simulink model "gm_IPCore_3Level_PWM"  (R2025b)
settings: Solver=VariableStepAuto  StartTime=0.0  StopTime=0.01  RelTol=1e-3
undefined symbols (not defined in the file or in its folder): f_Carrier, f_FPGA_clk, T_FPGA_clk
libraries: hdlsllib x3
settings Model: Creator=info  LastModifiedBy=info
settings OptimizationCC: BlockReduction=off  ConditionallyExecuteInputs=off  DefaultParameterBehavior=Inlined
settings DebuggingCC: AlgebraicLoopMsg=error  InheritedTsInSrcMsg=none  SingleTaskRateTransMsg=error
settings HardwareCC: ProdBitPerPointer=32.0  ProdBitPerSizeT=32.0  ProdBitPerPtrDiffT=32.0  ProdLargestAtomicFloat=None  ProdIntDivRoundTo=Undefined  ProdEndianess=Unspecified  ProdWordSize=32.0  ProdHWDeviceType=ASIC/FPGA->ASIC/FPGA  TargetBitPerPointer=64.0  TargetBitPerSizeT=64.0  TargetBitPerPtrDiffT=64.0  TargetLongLongMode=on  TargetIntDivRoundTo=Zero  TargetEndianess=LittleEndian  TargetWordSize=64.0  TargetHWDeviceType=Custom Processor->MATLAB Host Computer  ProdEqTarget=off

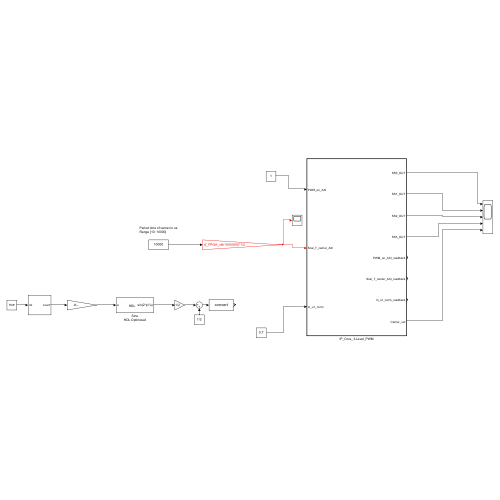
[thumbnail: Simulink's stored preview of the top-level diagram]
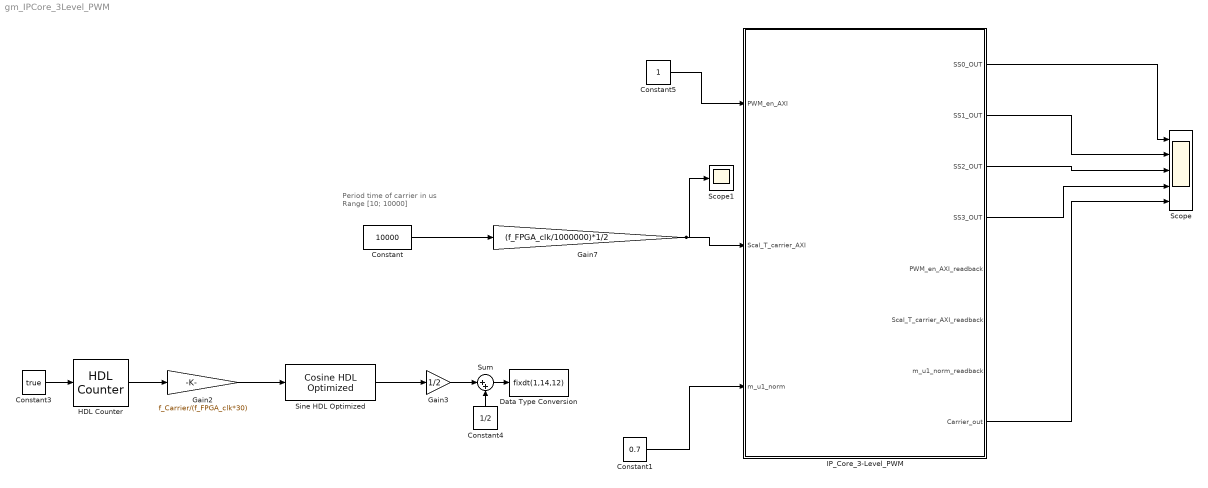
== system gm_IPCore_3Level_PWM ==
  note: Period time of carrier in us
      | Range [10; 10000]
  Constant : Constant  Value=10000  SampleTime=T_FPGA_clk
  Constant1 : Constant  Value=0.7  OutDataTypeStr=fixdt(1,14,12)  SampleTime=T_FPGA_clk
  Constant3 : Constant  Value=true  OutDataTypeStr=boolean  SampleTime=T_FPGA_clk
  Constant4 : Constant  Value=1/2  SampleTime=-1
  Constant5 : Constant  OutDataTypeStr=boolean  SampleTime=T_FPGA_clk
  Data Type Conversion : DataTypeConversion  OutDataTypeStr=fixdt(1,14,12)  SaturateOnIntegerOverflow=off  RndMeth=Floor
  Gain2 : Gain  Gain=f_Carrier/(f_FPGA_clk*30)
  Gain3 : Gain  Gain=1/2
  Gain7 : Gain  Gain=(f_FPGA_clk/1000000)*1/2  OutDataTypeStr=fixdt(0,25,0)
  HDL Counter : hdlsllib/Sources/HDL Counter  CountType=Free running  CountInit=0  CountStep=1  CountMax=25  CountFromType=Initial value  CountFrom=0  CountResetPort=off  CountLoadPort=off  CountEnbPort=off  CountDirPort=on  CountHitOutputPort=off  CountDataType=Unsigned  CountWordLen=20  CountFracLen=0  CountSampTime=1
  IP_Core_3-Level_PWM : Subsystem  TreatAsAtomicUnit=on
  Scope : Scope  NumInputPorts=5
      settings: ActiveDisplayYMinimum=-0.12499999999999997  ActiveDisplayYMaximum=1.125  DataLoggingVariableName=ScopeData2  DataLoggingSaveFormat=Array
  Scope1 : Scope
      settings: ActiveDisplayYMinimum=-2.0551334999999995E+6  ActiveDisplayYMaximum=1.85012015E+7  DataLoggingSaveFormat=Array
  Sine HDL Optimized : hdlsllib/Lookup Tables/Cosine HDL Optimized  OutputFormula=sin(2*pi*u)  NumDataPoints=64  TableDataTypeStr=fixdt(0,16,15)  SimulateLUTROMDelay=off
      settings: LibrarySourceBlock=|
      | hdlsllib/Lookup
      | Tables/Sine
      | HDL Optimized
  Sum : Sum  Inputs=|++
  wires:
  IP_Core_3-Level_PWM/8(Carrier_out) -> Scope/5
  Constant1/1 -> IP_Core_3-Level_PWM/3(m_u1_norm)
  IP_Core_3-Level_PWM/4(SS3_OUT) -> Scope/4
  IP_Core_3-Level_PWM/3(SS2_OUT) -> Scope/3
  IP_Core_3-Level_PWM/2(SS1_OUT) -> Scope/2
  IP_Core_3-Level_PWM/1(SS0_OUT) -> Scope/1
  Constant5/1 -> IP_Core_3-Level_PWM/1(PWM_en_AXI)
  Sum/1 -> Data Type Conversion/1
  Gain3/1 -> Sum/1
  Constant4/1 -> Sum/2
  Constant3/1 -> HDL Counter/1
  HDL Counter/1 -> Gain2/1
  Gain2/1 -> Sine HDL Optimized/1
  Sine HDL Optimized/1 -> Gain3/1
  Gain7/1 -> IP_Core_3-Level_PWM/2(Scal_T_carrier_AXI), Scope1/1
  Constant/1 -> Gain7/1

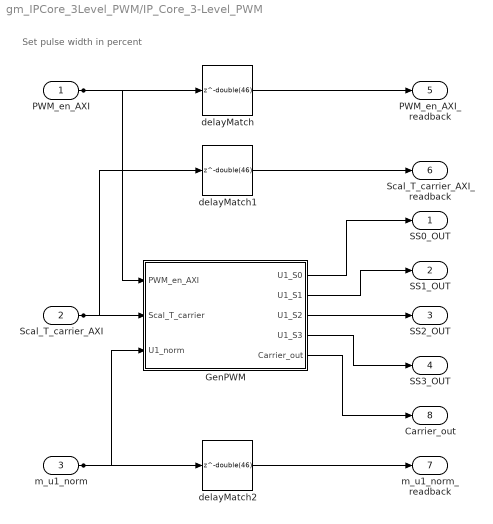
== system gm_IPCore_3Level_PWM/IP_Core_3-Level_PWM ==
  note: Set pulse width in percent
  PWM_en_AXI : Inport  OutDataTypeStr=boolean  PortDimensions=1  SampleTime=1e-08
  Scal_T_carrier_AXI : Inport  Port=2  OutDataTypeStr=fixdt(0, 25, 0)  PortDimensions=1  SampleTime=1e-08
  m_u1_norm : Inport  Port=3  OutDataTypeStr=fixdt(1, 14, 12)  PortDimensions=1  SampleTime=1e-08
  GenPWM : Subsystem
  delayMatch : Delay  DelayLength=double(46)  InitialCondition=0  SampleTime=1e-08
  delayMatch1 : Delay  DelayLength=double(46)  InitialCondition=0  SampleTime=1e-08
  delayMatch2 : Delay  DelayLength=double(46)  InitialCondition=0  SampleTime=1e-08
  SS0_OUT : Outport  SampleTime=1e-08  VectorParamsAs1DForOutWhenUnconnected=off
  SS1_OUT : Outport  Port=2  SampleTime=1e-08  VectorParamsAs1DForOutWhenUnconnected=off
  SS2_OUT : Outport  Port=3  SampleTime=1e-08  VectorParamsAs1DForOutWhenUnconnected=off
  SS3_OUT : Outport  Port=4  SampleTime=1e-08  VectorParamsAs1DForOutWhenUnconnected=off
  PWM_en_AXI_readback : Outport  Port=5  SampleTime=1e-08  VectorParamsAs1DForOutWhenUnconnected=off
  Scal_T_carrier_AXI_readback : Outport  Port=6  SampleTime=1e-08
  m_u1_norm_readback : Outport  Port=7  SampleTime=1e-08
  Carrier_out : Outport  Port=8  SampleTime=1e-08
  wires:
  PWM_en_AXI/1 -> GenPWM/1(PWM_en_AXI), delayMatch/1
  Scal_T_carrier_AXI/1 -> delayMatch1/1, GenPWM/2(Scal_T_carrier)
  delayMatch1/1 -> Scal_T_carrier_AXI_readback/1
  m_u1_norm/1 -> delayMatch2/1, GenPWM/3(U1_norm)
  delayMatch2/1 -> m_u1_norm_readback/1
  delayMatch/1 -> PWM_en_AXI_readback/1
  GenPWM/1(U1_S0) -> SS0_OUT/1
  GenPWM/2(U1_S1) -> SS1_OUT/1
  GenPWM/3(U1_S2) -> SS2_OUT/1
  GenPWM/4(U1_S3) -> SS3_OUT/1
  GenPWM/5(Carrier_out) -> Carrier_out/1

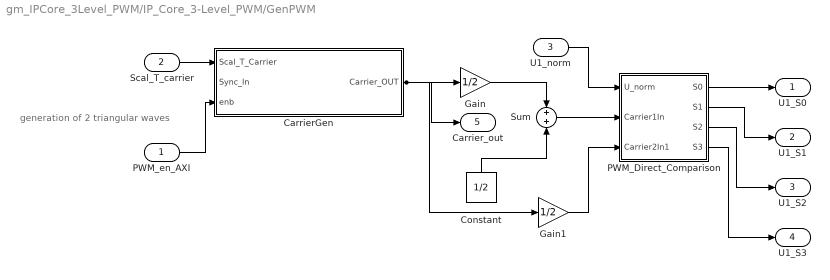
== system gm_IPCore_3Level_PWM/IP_Core_3-Level_PWM/GenPWM ==
  note: generation of 2 triangular waves
  PWM_en_AXI : Inport  OutDataTypeStr=boolean  PortDimensions=1  SampleTime=1e-08
  Scal_T_carrier : Inport  Port=2  OutDataTypeStr=fixdt(0, 25, 0)  PortDimensions=1  SampleTime=1e-08
  U1_norm : Inport  Port=3  OutDataTypeStr=fixdt(1, 14, 12)  PortDimensions=1  SampleTime=1e-08
  CarrierGen : Subsystem
  Constant : Constant  Value=1/2  OutDataTypeStr=fixdt(1,18,16)  SampleTime=T_FPGA_clk
  Gain : Gain  Gain=1/2  OutDataTypeStr=fixdt(1, 36, 33)
  Gain1 : Gain  Gain=1/2  OutDataTypeStr=fixdt(1, 36, 33)
  PWM_Direct_Comparison : Subsystem
  Sum : Sum  Inputs=+|+  OutDataTypeStr=fixdt(1, 37, 33)
  U1_S0 : Outport  SampleTime=1e-08
  U1_S1 : Outport  Port=2  SampleTime=1e-08
  U1_S2 : Outport  Port=3  SampleTime=1e-08
  U1_S3 : Outport  Port=4  SampleTime=1e-08
  Carrier_out : Outport  Port=5  SampleTime=1e-08
  wires:
  PWM_Direct_Comparison/1(S0) -> U1_S0/1
  CarrierGen/1(Carrier_OUT) -> Gain1/1, Gain/1, Carrier_out/1
  Scal_T_carrier/1 -> CarrierGen/1(Scal_T_Carrier)
  PWM_en_AXI/1 -> CarrierGen/3(enb)
  Sum/1 -> PWM_Direct_Comparison/2(Carrier1In)
  Gain/1 -> Sum/1
  U1_norm/1 -> PWM_Direct_Comparison/1(U_norm)
  Constant/1 -> Sum/2
  Gain1/1 -> PWM_Direct_Comparison/3(Carrier2In1)
  PWM_Direct_Comparison/2(S1) -> U1_S1/1
  PWM_Direct_Comparison/3(S2) -> U1_S2/1
  PWM_Direct_Comparison/4(S3) -> U1_S3/1

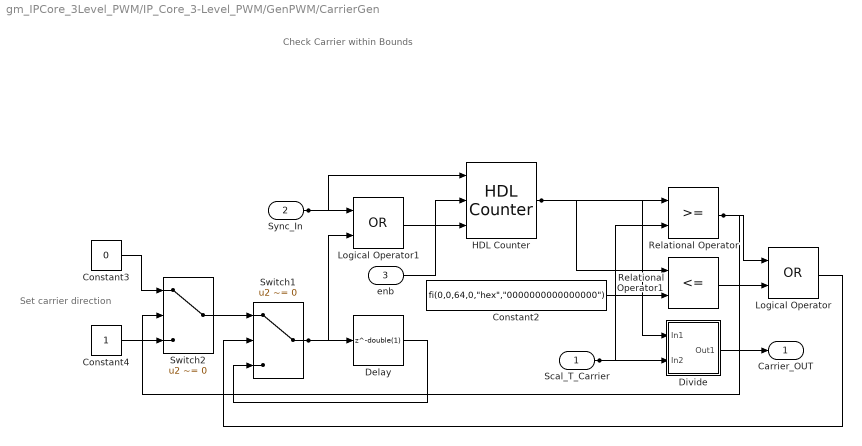
== system gm_IPCore_3Level_PWM/IP_Core_3-Level_PWM/GenPWM/CarrierGen ==
  note: Check Carrier within Bounds
  note: Set carrier direction
  Scal_T_Carrier : Inport  OutDataTypeStr=fixdt(0, 25, 0)  PortDimensions=1  SampleTime=1e-08
  Sync_In : Inport  Port=2  OutDataTypeStr=boolean  PortDimensions=1  SampleTime=1e-08
  enb : Inport  Port=3  OutDataTypeStr=boolean  PortDimensions=1  SampleTime=1e-08
  Constant2 : Constant  Value="fi(0,0,64,0,\"hex\",\"0000000000000000\")"  OutDataTypeStr=fixdt(0, 64, 0)  SampleTime=1e-08
  Constant3 : Constant  Value=0  OutDataTypeStr=boolean  SampleTime=1e-08
  Constant4 : Constant  OutDataTypeStr=boolean  SampleTime=1e-08
  Delay : Delay  DelayLength=double(1)  InitialCondition=0  SampleTime=1e-08
  Divide : Subsystem
  HDL Counter : hdlsllib/Sources/HDL Counter  CountType=Free running  CountInit=0  CountStep=1  CountMax=25  CountFromType=Initial value  CountFrom=0  CountResetPort=on  CountLoadPort=off  CountEnbPort=on  CountDirPort=on  CountHitOutputPort=off  CountDataType=Unsigned  CountWordLen=20  CountFracLen=0  CountSampTime=1
  Logical Operator : Logic  Operator=OR  AllPortsSameDT=off  OutDataTypeStr=boolean  SampleTime=1e-08
  Logical Operator1 : Logic  Operator=OR  AllPortsSameDT=off  OutDataTypeStr=boolean  SampleTime=1e-08
  Relational Operator : RelationalOperator  OutDataTypeStr=boolean  SampleTime=1e-08  InputSameDT=off
  Relational Operator1 : RelationalOperator  Operator=<=  OutDataTypeStr=boolean  SampleTime=1e-08  InputSameDT=off
  Switch1 : Switch  Criteria=u2 ~= 0  Threshold="fi(0,0,1,0,\"hex\",\"0\")"  OutDataTypeStr=boolean  SampleTime=1e-08  SaturateOnIntegerOverflow=off  InputSameDT=off
  Switch2 : Switch  Criteria=u2 ~= 0  Threshold="fi(0,0,1,0,\"hex\",\"0\")"  OutDataTypeStr=boolean  SampleTime=1e-08  SaturateOnIntegerOverflow=off  InputSameDT=off
  Carrier_OUT : Outport  SampleTime=1e-08
  wires:
  Constant3/1 -> Switch2/1
  Sync_In/1 -> HDL Counter/1, Logical Operator1/1
  Constant4/1 -> Switch2/3
  Switch2/1 -> Switch1/1
  Switch1/1 -> Delay/1, Logical Operator1/2
  Delay/1 -> Switch1/3
  Logical Operator1/1 -> HDL Counter/3
  enb/1 -> HDL Counter/2
  HDL Counter/1 -> Relational Operator/1, Relational Operator1/1, Divide/1(In1)
  Constant2/1 -> Relational Operator1/2
  Scal_T_Carrier/1 -> Relational Operator/2, Divide/2(In2)
  Relational Operator/1 -> Switch2/2, Logical Operator/1
  Relational Operator1/1 -> Logical Operator/2
  Divide/1(Out1) -> Carrier_OUT/1
  Logical Operator/1 -> Switch1/2

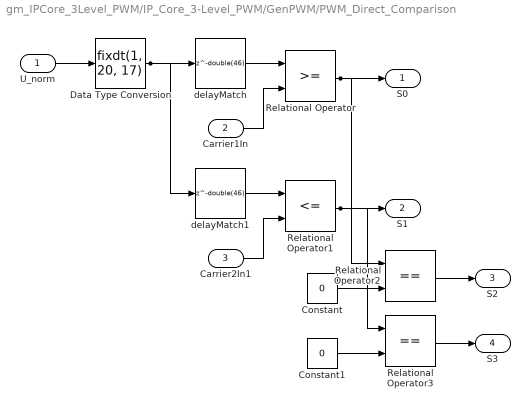
== system gm_IPCore_3Level_PWM/IP_Core_3-Level_PWM/GenPWM/PWM_Direct_Comparison ==
  U_norm : Inport  OutDataTypeStr=fixdt(1, 14, 12)  PortDimensions=1  SampleTime=1e-08
  Carrier1In : Inport  Port=2  OutDataTypeStr=fixdt(1, 37, 33)  PortDimensions=1  SampleTime=1e-08
  Carrier2In1 : Inport  Port=3  OutDataTypeStr=fixdt(1, 36, 33)  PortDimensions=1  SampleTime=1e-08
  Constant : Constant  Value=0  OutDataTypeStr=boolean  SampleTime=1e-08
  Constant1 : Constant  Value=0  OutDataTypeStr=boolean  SampleTime=1e-08
  Data Type Conversion : DataTypeConversion  OutDataTypeStr=fixdt(1, 20, 17)  RndMeth=Nearest  SampleTime=1e-08  SaturateOnIntegerOverflow=off
  Relational Operator : RelationalOperator  OutDataTypeStr=boolean  SampleTime=1e-08  InputSameDT=off
  Relational Operator1 : RelationalOperator  Operator=<=  OutDataTypeStr=boolean  SampleTime=1e-08  InputSameDT=off
  Relational Operator2 : RelationalOperator  Operator===  OutDataTypeStr=boolean  SampleTime=1e-08  InputSameDT=off
  Relational Operator3 : RelationalOperator  Operator===  OutDataTypeStr=boolean  SampleTime=1e-08  InputSameDT=off
  delayMatch : Delay  DelayLength=double(46)  InitialCondition=0  SampleTime=1e-08
  delayMatch1 : Delay  DelayLength=double(46)  InitialCondition=0  SampleTime=1e-08
  S0 : Outport  SampleTime=1e-08
  S1 : Outport  Port=2  SampleTime=1e-08
  S2 : Outport  Port=3  SampleTime=1e-08
  S3 : Outport  Port=4  SampleTime=1e-08
  wires:
  Relational Operator/1 -> Relational Operator2/1, S0/1
  U_norm/1 -> Data Type Conversion/1
  Data Type Conversion/1 -> delayMatch1/1, delayMatch/1
  Carrier2In1/1 -> Relational Operator1/2
  delayMatch/1 -> Relational Operator/1
  Carrier1In/1 -> Relational Operator/2
  delayMatch1/1 -> Relational Operator1/1
  Relational Operator1/1 -> Relational Operator3/1, S1/1
  Constant/1 -> Relational Operator2/2
  Constant1/1 -> Relational Operator3/2
  Relational Operator2/1 -> S2/1
  Relational Operator3/1 -> S3/1

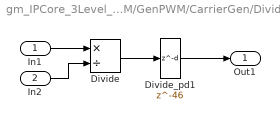
== system gm_IPCore_3Level_PWM/IP_Core_3-Level_PWM/GenPWM/CarrierGen/Divide ==
  In1 : Inport
  In2 : Inport  Port=2
  Divide : Product  Inputs=*/  OutDataTypeStr=fixdt(1,18,16)  RndMeth=Zero  SaturateOnIntegerOverflow=on
  Divide_pd1 : Delay  DelayLength=46
  Out1 : Outport
  wires:
  In1/1 -> Divide/1
  In2/1 -> Divide/2
  Divide/1 -> Divide_pd1/1
  Divide_pd1/1 -> Out1/1
